simulink library "tethers_cl"  (R2018b)
settings: Solver=VariableStepAuto  StartTime=0.0  StopTime=10.0  RelTol=1e-3
undefined symbols (not defined in the file or in its folder): ini_Ri_o, ini_Vi_o, N, thr
libraries: tetherBuoyancyAndWeight_ul x1, tetherDragForce_ul x1, tetherInternalForces_ul x1
settings Model: Creator=mcobb  LastModifiedBy=mcobb

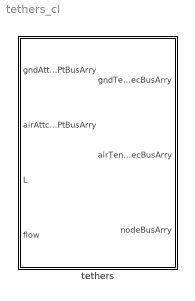
== system tethers_cl ==
  tethers : Subsystem  mask{thr=thr}
      mask prompts: thr "Tether parameter structure"
      mask help:
      | Tether parameters structure must have the form
      | thr(i).N                = sim_param.N;
      | thr(i).diameter         = sim_param.tether_param.tether_diameter(i);
      | thr(i).youngsMod        = sim_param.tether_param.tether_youngs;
      | thr(i).density          = sim_param.tether_param.tether_density+ sim_param.env_param.density;
      | thr(i).dragCoeff        = sim_param.tether_param.CD_cylinder;
      | thr(i).dampingRatio     = sim_param.tether_param.damping_ratio;
      | thr(i).fluidDensity     = sim_param.env_param.density;
      | thr(i).gravAccel        = sim_param.env_param.grav;
      | thr(i).vehicleMass      = sim_param.geom_param.mass;
      | thr(i).initVhclAttchPt  = ini_Rcm_o + rotation_sequence(ini_euler_ang)*R1n_cm;
      | thr(i).initGndStnAttchPt  = gnd_station + R11_g;
      mask init:
      | tether_init

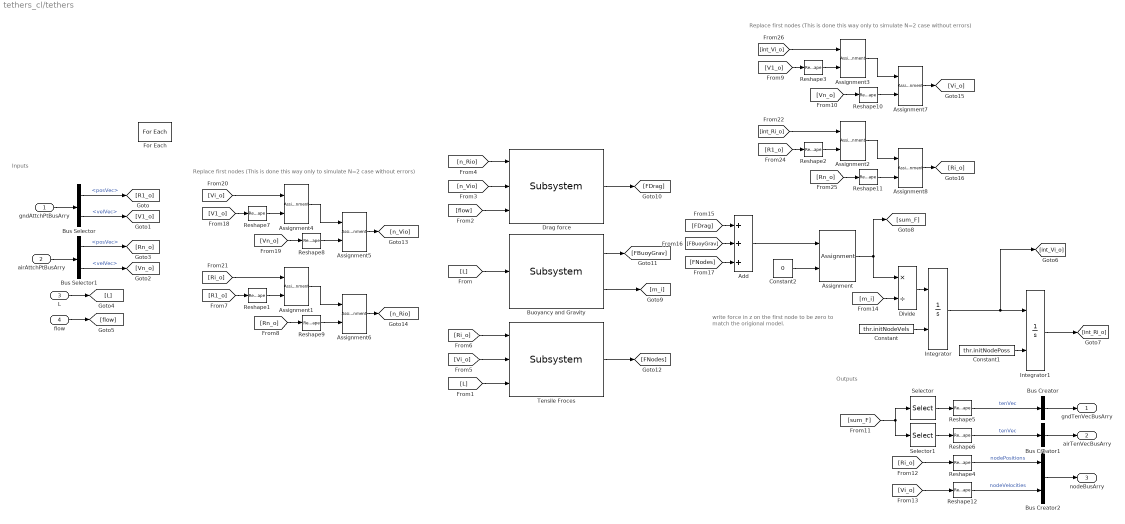
== system tethers_cl/tethers ==
  note: Replace first nodes (This is done this way only to simulate N=2 case
      | without errors)
  note: Inputs
  note: Outputs
  note: Replace first nodes (This is done this way only to simulate N=2 case
      | without errors)
  note: write force in z on the first node to be zero
      | to match the origional model.
  gndAttchPtBusArry : Inport  OutDataTypeStr=Bus: thrAttachPtKinematicsBus  Partition=on  PartitionDimension=1  PartitionWidth=1  PartitionOffset=0
  airAttchPtBusArry : Inport  Port=2  OutDataTypeStr=Bus: thrAttachPtKinematicsBus  Partition=on  PartitionDimension=1  PartitionWidth=1  PartitionOffset=0
  L : Inport  Port=3  Partition=on  PartitionDimension=1  PartitionWidth=1  PartitionOffset=0
  flow : Inport  Port=4
  Add : Sum  Inputs=+++
  Assignment : Assignment  NumberOfDimensions=2  DiagnosticForDimensions=Warning  IndexOptions=Index vector (dialog),Index vector (dialog)  Indices=3,1  OutputSizes=1,1
  Assignment{1..4} (4 alike) : Assignment  NumberOfDimensions=2  DiagnosticForDimensions=Warning  IndexOptions=Assign all,Index vector (dialog)  Indices=1,1  OutputSizes=1,1
  Assignment{5..8} (4 alike) : Assignment  NumberOfDimensions=2  DiagnosticForDimensions=Warning  IndexOptions=Assign all,Index vector (dialog)  Indices=1,N  OutputSizes=1,1
  Buoyancy and Gravity : tetherBuoyancyAndWeight_ul/Subsystem  N=thr.N  dia_t=thr.diameter  rho_fluid=thr.fluidDensity  rho_tether=thr.density  g=thr.gravAccel
  Bus Creator : BusCreator  Inputs=1  OutDataTypeStr=Bus: thrTenVecBus  NonVirtualBus=on
  Bus Creator1 : BusCreator  Inputs=1  OutDataTypeStr=Bus: thrTenVecBus  NonVirtualBus=on
  Bus Creator2 : BusCreator  Inputs=2
  Bus Selector : BusSelector  OutputSignals=posVec,velVec
  Bus Selector1 : BusSelector  OutputSignals=posVec,velVec
  Constant : Constant  Value=thr.initNodeVels
  Constant1 : Constant  Value=thr.initNodePoss
  Constant2 : Constant  Value=0
  Divide : Product  Inputs=*/
  Drag force : tetherDragForce_ul/Subsystem  Cd=thr.dragCoeff  rho_fluid=thr.fluidDensity  dia_t=thr.diameter
  For Each : ForEach  DisableCoverage=on  IterateSubsysMaskParameter=on  SubsysMaskParameterIterationDimension=2  IndexMode=One-based
  Integrator : Integrator  InitialConditionSource=external  InitialCondition=ini_Vi_o
  Integrator1 : Integrator  InitialConditionSource=external  InitialCondition=ini_Ri_o
  Reshape{1..12} (12 alike) : Reshape  OutputDimensionality=Column vector (2-D)
  Selector : Selector  NumberOfDimensions=2  InputPortWidth=3  IndexOptions=Select all,Index vector (dialog)  Indices=[1],1  OutputSizes=1,1
  Selector1 : Selector  NumberOfDimensions=2  InputPortWidth=3  IndexOptions=Select all,Index vector (dialog)  Indices=[N],N  OutputSizes=1,1
  Tensile Froces : tetherInternalForces_ul/Subsystem  N=thr.N  E=thr.youngsMod  dia_t=thr.diameter  mass=thr.vehicleMass  zeta=thr.dampingRatio
  gndTenVecBusArry : Outport  ConcatenationDimension=1
  airTenVecBusArry : Outport  Port=2  ConcatenationDimension=1
  nodeBusArry : Outport  Port=3  ConcatenationDimension=1
  wires:
  Constant2/1 -> Assignment/2
  Add/1 -> Assignment/1
  Assignment/1 -> Divide/1, [sum_F]
  Reshape2/1 -> Assignment2/2
  Assignment8/1 -> [Ri_o]
  Reshape10/1 -> Assignment7/2
  [int_Ri_o] -> Assignment2/1
  Assignment2/1 -> Assignment8/1
  Assignment7/1 -> [Vi_o]
  [Rn_o] -> Reshape11/1
  [Vn_o] -> Reshape10/1
  [R1_o] -> Reshape2/1
  [int_Vi_o] -> Assignment3/1
  Reshape11/1 -> Assignment8/2
  Assignment3/1 -> Assignment7/1
  Reshape3/1 -> Assignment3/2
  [V1_o] -> Reshape3/1
  Integrator1/1 -> [int_Ri_o]
  Reshape9/1 -> Assignment6/2
  Reshape1/1 -> Assignment1/2
  [Ri_o] -> Assignment1/1
  Assignment6/1 -> [n_Rio]
  [Rn_o] -> Reshape9/1
  [R1_o] -> Reshape1/1
  Assignment1/1 -> Assignment6/1
  [n_Vio] -> Drag force/2
  Assignment5/1 -> [n_Vio]
  Assignment4/1 -> Assignment5/1
  Reshape8/1 -> Assignment5/2
  [Vn_o] -> Reshape8/1
  [Vi_o] -> Assignment4/1
  [V1_o] -> Reshape7/1
  Reshape7/1 -> Assignment4/2
  [FNodes] -> Add/3
  [FDrag] -> Add/1
  [FBuoyGrav] -> Add/2
  [m_i] -> Divide/2
  Buoyancy and Gravity/2 -> [m_i]
  Constant1/1 -> Integrator1/2
  Constant/1 -> Integrator/2
  Reshape5/1 -> Bus Creator/1  "tenVec"
  Selector/1 -> Reshape5/1
  Reshape6/1 -> Bus Creator1/1  "tenVec"
  Selector1/1 -> Reshape6/1
  [Vi_o] -> Reshape12/1
  [Ri_o] -> Reshape4/1
  [sum_F] -> Selector1/1, Selector/1
  Integrator/1 -> Integrator1/1, [int_Vi_o]
  [Ri_o] -> Tensile Froces/1
  [Vi_o] -> Tensile Froces/2
  [n_Rio] -> Drag force/1
  Divide/1 -> Integrator/1
  Tensile Froces/1 -> [FNodes]
  Drag force/1 -> [FDrag]
  Buoyancy and Gravity/1 -> [FBuoyGrav]
  [flow] -> Drag force/3
  [L] -> Tensile Froces/3
  [L] -> Buoyancy and Gravity/1
  flow/1 -> [flow]
  L/1 -> [L]
  gndAttchPtBusArry/1 -> Bus Selector/1
  Bus Selector1/1 -> [Rn_o]  "<posVec>"
  Bus Selector/1 -> [R1_o]  "<posVec>"
  Bus Selector/2 -> [V1_o]  "<velVec>"
  Bus Selector1/2 -> [Vn_o]  "<velVec>"
  Reshape4/1 -> Bus Creator2/1  "nodePositions"
  Reshape12/1 -> Bus Creator2/2  "nodeVelocities"
  Bus Creator/1 -> gndTenVecBusArry/1
  Bus Creator1/1 -> airTenVecBusArry/1
  Bus Creator2/1 -> nodeBusArry/1
  airAttchPtBusArry/1 -> Bus Selector1/1
